simulink model "PID_model"  (R2020a)
settings: Solver=VariableStepAuto  StartTime=0.0  StopTime=10  RelTol=1e-3
values from neighbouring files (symbols this model uses):
  A = [0 0 0 1 0 0 0 0 0 0 0 0 ... (first row only)    [quadrotor_parameters.m]
  B = [0 0 0 0 ... (first row only)    [quadrotor_parameters.m]
  kf = 9.8e-6    (= 9.8e-06)    [quadrotor_parameters.m]
  km = 1.6e-7    (= 1.6e-07)    [quadrotor_parameters.m]
  w1 = 100    [quadrotor_parameters.m]
  w2 = 100    [quadrotor_parameters.m]
  w3 = 100    [quadrotor_parameters.m]
  w4 = 100    [quadrotor_parameters.m]
libraries: simulink x6
settings Model: Creator=Dr.Saraf  LastModifiedBy=Dr.Saraf
settings DataIOCC: ReturnWorkspaceOutputs=off
settings DebuggingCC: ArithmeticOperatorsInVariantConditions=warning
settings SFSimCC: SimUseLocalCustomCode=off  CustomCodeUndefinedFunction=UseInterfaceOnly
settings RTWCC: RTWUseLocalCustomCode=off
settings CodeAppCC: StateflowObjectComments=on

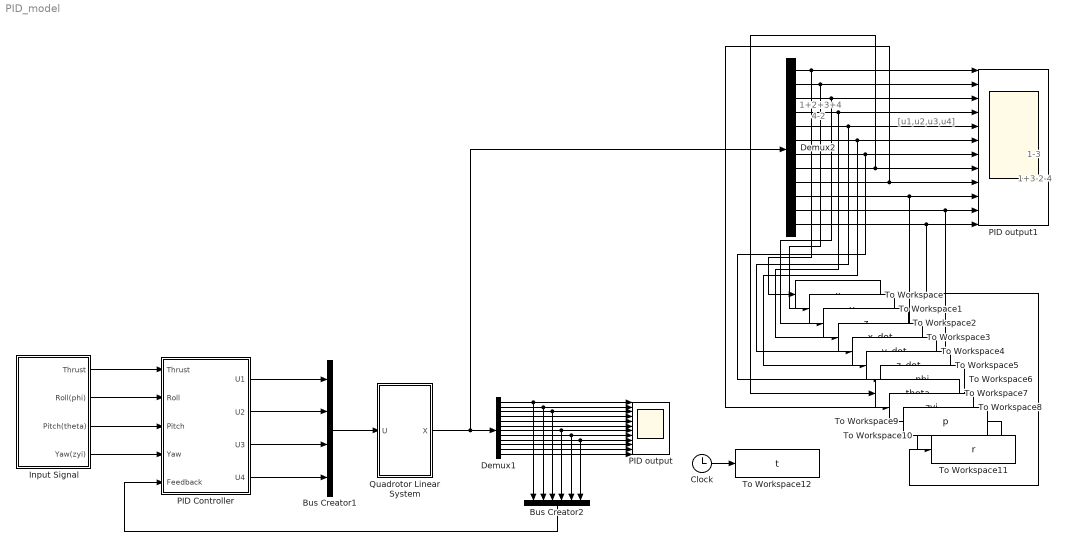
== system PID_model ==
  note: [u1,u2,u3,u4]
  note: 1+2+3+4
  note: 1+3-2-4
  note: 1-3
  note: 4-2
  Bus Creator1 : BusCreator  Inputs=4
  Bus Creator2 : BusCreator  Inputs=6
  Clock : Clock
  Demux1 : Demux  Outputs=12
  Demux2 : Demux  Outputs=12
  Input Signal : Subsystem
  PID Controller : Subsystem
  "PID output " : Scope  NumInputPorts=12
  "PID output1 " : Scope  NumInputPorts=12
  Quadrotor Linear System : Subsystem
  To Workspace : ToWorkspace  VariableName=x  SampleTime=0.1
  To Workspace1 : ToWorkspace  VariableName=y  SampleTime=0.1
  To Workspace10 : ToWorkspace  VariableName=q  SampleTime=0.001
  To Workspace11 : ToWorkspace  VariableName=r  SampleTime=0.001
  To Workspace12 : ToWorkspace  VariableName=t  SampleTime=0.001
  To Workspace2 : ToWorkspace  VariableName=z  SampleTime=0.1
  To Workspace3 : ToWorkspace  VariableName=x_dot  SampleTime=0.1
  To Workspace4 : ToWorkspace  VariableName=y_dot  SampleTime=0.1
  To Workspace5 : ToWorkspace  VariableName=z_dot  SampleTime=0.1
  To Workspace6 : ToWorkspace  VariableName=phi  SampleTime=0.001
  To Workspace7 : ToWorkspace  VariableName=theta  SampleTime=0.001
  To Workspace8 : ToWorkspace  VariableName=zyi  SampleTime=0.001
  To Workspace9 : ToWorkspace  VariableName=p  SampleTime=0.001
  wires:
  Demux1/5 -> "PID output "/5
  Demux1/11 -> "PID output "/11
  Demux1/12 -> "PID output "/12
  Demux1/4 -> "PID output "/4
  Demux1/10 -> "PID output "/10
  Demux1/6 -> "PID output "/6
  Demux1/1 -> "PID output "/1, Bus Creator2/1
  Demux1/9 -> "PID output "/9, Bus Creator2/6
  Demux1/7 -> "PID output "/7, Bus Creator2/4
  Demux1/3 -> "PID output "/3, Bus Creator2/3
  Demux1/8 -> "PID output "/8, Bus Creator2/5
  Demux1/2 -> "PID output "/2, Bus Creator2/2
  Bus Creator1/1 -> Quadrotor Linear System/1(U)
  Quadrotor Linear System/1(X) -> Demux2/1, Demux1/1
  Input Signal/1(Thrust) -> PID Controller/1(Thrust)
  Input Signal/2(Roll(phi)) -> PID Controller/2(Roll)
  Input Signal/3(Pitch(theta)) -> PID Controller/3(Pitch)
  Input Signal/4(Yaw(zyi)) -> PID Controller/4(Yaw)
  Bus Creator2/1 -> PID Controller/5(Feedback)
  PID Controller/1(U1) -> Bus Creator1/1
  PID Controller/2(U2) -> Bus Creator1/2
  PID Controller/3(U3) -> Bus Creator1/3
  PID Controller/4(U4) -> Bus Creator1/4
  Clock/1 -> To Workspace12/1
  Demux2/11 -> To Workspace10/1, "PID output1 "/11
  Demux2/5 -> To Workspace4/1, "PID output1 "/5
  Demux2/8 -> To Workspace7/1, "PID output1 "/8
  Demux2/10 -> To Workspace9/1, "PID output1 "/10
  Demux2/1 -> To Workspace/1, "PID output1 "/1
  Demux2/12 -> To Workspace11/1, "PID output1 "/12
  Demux2/3 -> To Workspace2/1, "PID output1 "/3
  Demux2/6 -> To Workspace5/1, "PID output1 "/6
  Demux2/9 -> To Workspace8/1, "PID output1 "/9
  Demux2/2 -> To Workspace1/1, "PID output1 "/2
  Demux2/4 -> To Workspace3/1, "PID output1 "/4
  Demux2/7 -> To Workspace6/1, "PID output1 "/7

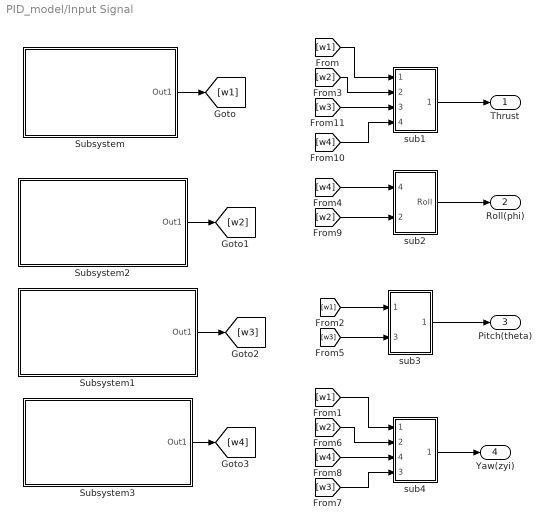
== system PID_model/Input Signal ==
  Subsystem : Subsystem
  Subsystem1 : Subsystem
  Subsystem2 : Subsystem
  Subsystem3 : Subsystem
  sub1 : Subsystem
  "sub2 " : Subsystem
  "sub3 " : Subsystem
  sub4 : Subsystem
  Thrust : Outport
  Roll(phi) : Outport  Port=2
  Pitch(theta) : Outport  Port=3
  Yaw(zyi) : Outport  Port=4
  wires:
  [w4] -> sub1/4(4)
  [w3] -> sub1/3(3)
  [w2] -> sub1/2(2)
  [w1] -> sub4/1(1)
  [w4] -> sub4/3("4 ")
  [w3] -> sub4/4("3 ")
  [w1] -> "sub3 "/1(1)
  [w4] -> "sub2 "/1(4)
  [w3] -> "sub3 "/2(3)
  [w1] -> sub1/1(1)
  [w2] -> sub4/2(2)
  [w2] -> "sub2 "/2(2)
  "sub2 "/1(Roll) -> Roll(phi)/1
  sub1/1(Thrust) -> Thrust/1
  sub4/1(Yaw) -> Yaw(zyi)/1
  "sub3 "/1(Pitch) -> Pitch(theta)/1
  Subsystem1/1(Out1) -> [w3]
  Subsystem/1(Out1) -> [w1]
  Subsystem2/1(Out1) -> [w2]
  Subsystem3/1(Out1) -> [w4]

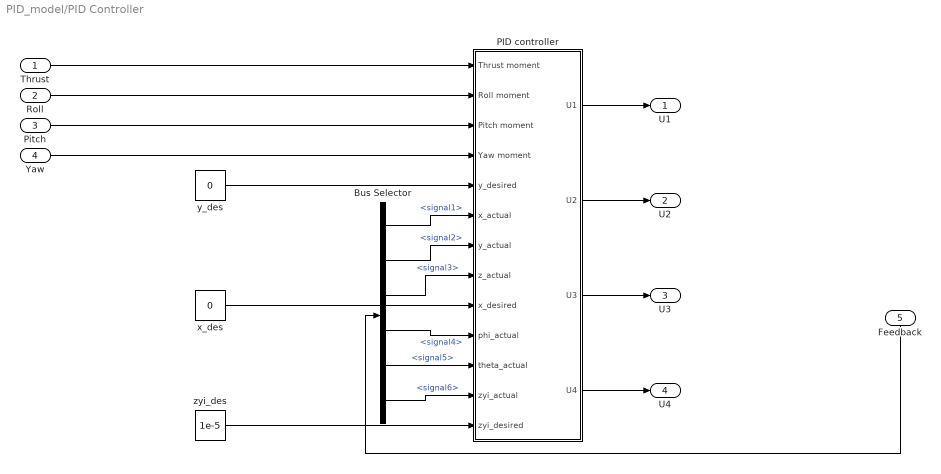
== system PID_model/PID Controller ==
  Thrust : Inport
  Roll : Inport  Port=2
  Pitch : Inport  Port=3
  Yaw : Inport  Port=4
  Feedback : Inport  Port=5
  Bus Selector : BusSelector  OutputSignals=signal1,signal2,signal3,signal4,signal5,signal6
  PID controller : Subsystem
  x_des : Constant  Value=0
  y_des : Constant  Value=0
  zyi_des : Constant  Value=1e-5
  U1 : Outport
  U2 : Outport  Port=2
  U3 : Outport  Port=3
  U4 : Outport  Port=4
  wires:
  Bus Selector/1 -> PID controller/6(x_actual)  "<signal1>"
  Thrust/1 -> PID controller/1(Thrust moment)
  Roll/1 -> PID controller/2(Roll moment)
  PID controller/3("U3 ") -> U3/1
  Bus Selector/2 -> PID controller/7(y_actual)  "<signal2>"
  x_des/1 -> PID controller/9(x_desired)
  zyi_des/1 -> PID controller/13(zyi_desired)
  Bus Selector/3 -> PID controller/8(z_actual)  "<signal3>"
  Bus Selector/6 -> PID controller/12(zyi_actual)  "<signal6>"
  Feedback/1 -> Bus Selector/1
  y_des/1 -> PID controller/5(y_desired)
  PID controller/2(U2) -> U2/1
  Yaw/1 -> PID controller/4(Yaw moment)
  Bus Selector/4 -> PID controller/10(phi_actual)  "<signal4>"
  PID controller/4(U4) -> U4/1
  Pitch/1 -> PID controller/3(Pitch moment)
  PID controller/1(U1) -> U1/1
  Bus Selector/5 -> PID controller/11(theta_actual)  "<signal5>"

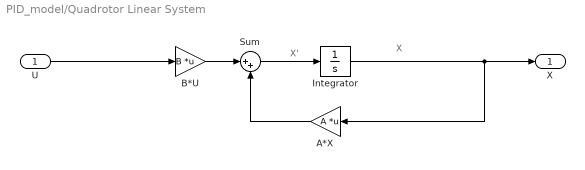
== system PID_model/Quadrotor Linear System ==
  note: X'
  note: X
  U : Inport
  A*X : Gain  Gain=A  Multiplication=Matrix(K*u)
  B*U : Gain  Gain=B  Multiplication=Matrix(K*u)
  Integrator : Integrator  InitialCondition=[1,1,1,1,1,1,1,1,1,1,1,1]
  Sum : Sum  Inputs=|++
  X : Outport
  wires:
  Integrator/1 -> X/1, A*X/1
  B*U/1 -> Sum/1
  Sum/1 -> Integrator/1
  A*X/1 -> Sum/2
  U/1 -> B*U/1

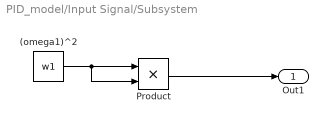
== system PID_model/Input Signal/Subsystem ==
  (omega1)^2 : Constant  Value=w1
  Product : Product
  Out1 : Outport
  wires:
  (omega1)^2/1 -> Product/2, Product/1
  Product/1 -> Out1/1

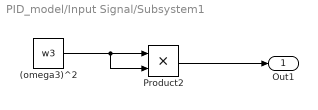
== system PID_model/Input Signal/Subsystem1 ==
  (omega3)^2 : Constant  Value=w3
  Product2 : Product
  Out1 : Outport
  wires:
  (omega3)^2/1 -> Product2/2, Product2/1
  Product2/1 -> Out1/1

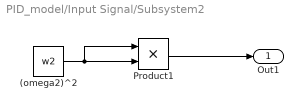
== system PID_model/Input Signal/Subsystem2 ==
  (omega2)^2 : Constant  Value=w2
  Product1 : Product
  Out1 : Outport
  wires:
  (omega2)^2/1 -> Product1/1, Product1/2
  Product1/1 -> Out1/1

== system PID_model/Input Signal/Subsystem3 ==
  (omega4)^2 : Constant  Value=w4
  Product3 : Product
  Out1 : Outport
  wires:
  (omega4)^2/1 -> Product3/2, Product3/1
  Product3/1 -> Out1/1

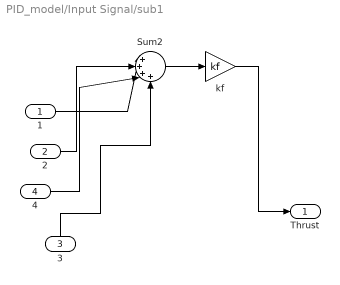
== system PID_model/Input Signal/sub1 ==
  1 : Inport
  2 : Inport  Port=2
  3 : Inport  Port=3
  4 : Inport  Port=4
  Sum2 : Sum  Inputs=|++++
  kf : Gain  Gain=kf
  Thrust : Outport
  wires:
  kf/1 -> Thrust/1
  Sum2/1 -> kf/1
  1/1 -> Sum2/1
  2/1 -> Sum2/2
  3/1 -> Sum2/4
  4/1 -> Sum2/3

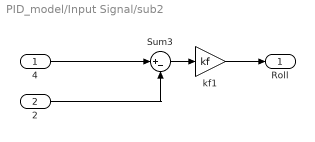
== system PID_model/Input Signal/sub2  ==
  4 : Inport
  2 : Inport  Port=2
  Sum3 : Sum  Inputs=|+-
  kf1 : Gain  Gain=kf
  Roll : Outport
  wires:
  kf1/1 -> Roll/1
  Sum3/1 -> kf1/1
  4/1 -> Sum3/1
  2/1 -> Sum3/2

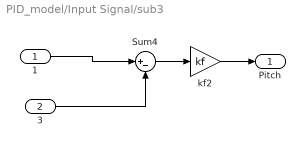
== system PID_model/Input Signal/sub3  ==
  1 : Inport
  3 : Inport  Port=2
  Sum4 : Sum  Inputs=|+-
  kf2 : Gain  Gain=kf
  Pitch : Outport
  wires:
  3/1 -> Sum4/2
  1/1 -> Sum4/1
  Sum4/1 -> kf2/1
  kf2/1 -> Pitch/1

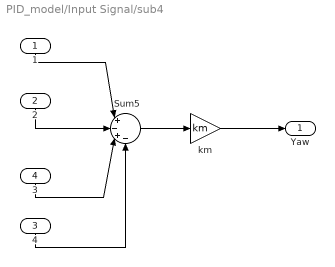
== system PID_model/Input Signal/sub4 ==
  1 : Inport
  2 : Inport  Port=2
  "4 " : Inport  Port=3
  "3 " : Inport  Port=4
  Sum5 : Sum  Inputs=|+-+-
  km : Gain  Gain=km
  Yaw : Outport
  wires:
  Sum5/1 -> km/1
  km/1 -> Yaw/1
  "3 "/1 -> Sum5/3
  2/1 -> Sum5/2
  "4 "/1 -> Sum5/4
  1/1 -> Sum5/1

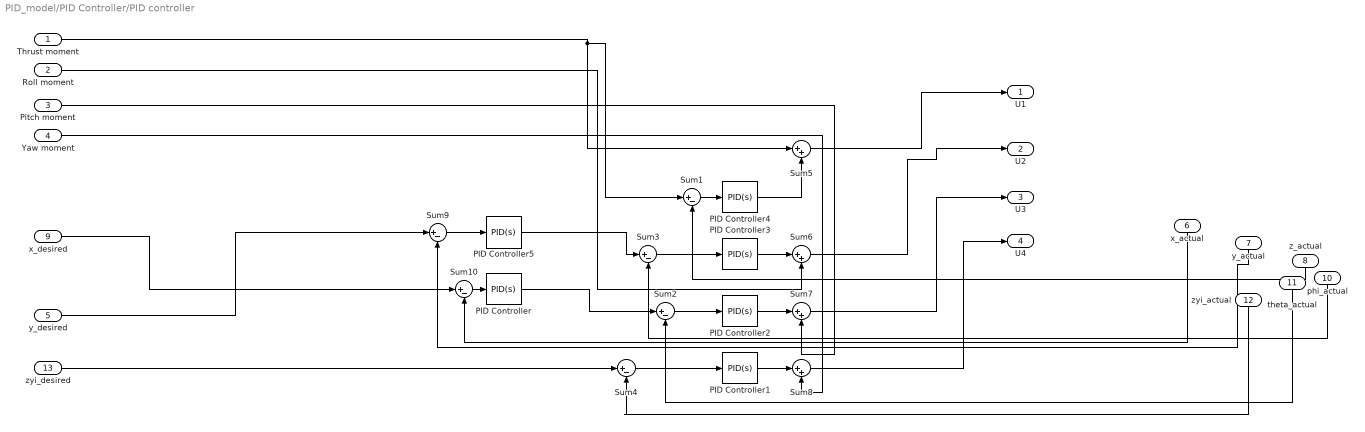
== system PID_model/PID Controller/PID controller ==
  Thrust moment : Inport
  Roll moment : Inport  Port=2
  Pitch moment : Inport  Port=3
  Yaw moment : Inport  Port=4
  y_desired : Inport  Port=5
  x_actual : Inport  Port=6
  y_actual : Inport  Port=7
  z_actual : Inport  Port=8
  x_desired : Inport  Port=9
  phi_actual : Inport  Port=10
  theta_actual : Inport  Port=11
  zyi_actual : Inport  Port=12
  zyi_desired : Inport  Port=13
  PID Controller : simulink/Continuous/PID Controller  Controller=PID  Form=Parallel  TimeDomain=Continuous-time  UseExternalTs=off  SampleTime=-1  IntegratorMethod=Forward Euler  FilterMethod=Forward Euler  ControllerParametersSource=internal  P=2.93760850093011  I=0.0320571710777629  D=4.86506551746036  UseFilter=on  N=2.18607719154356  TunerSelectOption=Transfer Function Based (PID Tuner App)  InitialConditionSource=internal  InitialConditionForIntegrator=0  InitialConditionForFilter=0  DifferentiatorICPrevScaledInput=0  ExternalReset=none  TrackingMode=off  Kt=1  LimitOutput=off  UpperSaturationLimit=inf  LowerSaturationLimit=-inf  LinearizeAsGain=on  AntiWindupMode=none  Kb=1  POutMin=[]  POutMax=[]  IOutMin=[]  IOutMax=[]  DOutMin=[]  DOutMax=[]  NOutMin=[]  NOutMax=[]  SumOutMin=[]  SumOutMax=[]  SaturationOutMin=[]  SaturationOutMax=[]  PParamMin=[]  PParamMax=[]  IParamMin=[]  IParamMax=[]  DParamMin=[]  DParamMax=[]  NParamMin=[]  NParamMax=[]  KbParamMin=[]  KbParamMax=[]  KtParamMin=[]  KtParamMax=[]  KbOutMin=[]  KbOutMax=[]  KtOutMin=[]  KtOutMax=[]  IntegratorOutMin=[]  IntegratorOutMax=[]  FilterOutMin=[]  FilterOutMax=[]  SumI1OutMin=[]  SumI1OutMax=[]  SumI2OutMin=[]  SumI2OutMax=[]  SumI3OutMin=[]  SumI3OutMax=[]  SumI4OutMin=[]  SumI4OutMax=[]  SumDOutMin=[]  SumDOutMax=[]  DifferentiatorOutMin=[]  DifferentiatorOutMax=[]  FilterDiffOutCoefMin=[]  FilterDiffOutCoefMax=[]  ReciprocalOutMin=[]  ReciprocalOutMax=[]  SumDenOutMin=[]  SumDenOutMax=[]  SumNumOutMin=[]  SumNumOutMax=[]  DivideOutMin=[]  DivideOutMax=[]  UdiffTsProdOutMin=[]  UdiffTsProdOutMax=[]  NTsProdOutMin=[]  NTsProdOutMax=[]  UintegralTsProdOutMin=[]  UintegralTsProdOutMax=[]  UngainTsProdOutMin=[]  UngainTsProdOutMax=[]  IntegratorContinuousStateAttributes=''  IntegratorStateMustResolveToSignalObject=off  IntegratorRTWStateStorageClass=Auto  FilterContinuousStateAttributes=''  FilterStateMustResolveToSignalObject=off  FilterRTWStateStorageClass=Auto  ParallelPVariant=InternalParameters  IdealPVariant=Disabled  IVariant=InternalParameters  DVariant=InternalParameters  IntegratorVariant=Continuous  SatVariant=Disabled  AWVariant=Passthrough  PCopyVariant=Disabled  TRVariant=Disabled  FdbkBlocksVariant=Forward  IdealPFdbkVariant=Disabled  SatFdbkVariant=Disabled  DerivativeFilterVariant=ContFilter  NVariant=InternalParameters  NCopyVariant=Disabled  FilterICVariant=InternalICsFilter  IntegratorICVariant=InternalICs  ExternalResetVariant=Disabled  TRSumVariant=Passthrough  SumFdbkVariant=Disabled  SumVariant=Sum_PID  TsampFilterVariant=InternalTs  TsampNgainVariant=Passthrough  TsampIntegralVariant=Passthrough
  PID Controller1 : simulink/Continuous/PID Controller  Controller=PID  Form=Parallel  TimeDomain=Continuous-time  UseExternalTs=off  SampleTime=-1  IntegratorMethod=Forward Euler  FilterMethod=Forward Euler  ControllerParametersSource=internal  P=0.0131233252055703  I=0.000765605460811457  D=0.0499808607427746  UseFilter=on  N=1142.8279760416  TunerSelectOption=Transfer Function Based (PID Tuner App)  InitialConditionSource=internal  InitialConditionForIntegrator=0  InitialConditionForFilter=0  DifferentiatorICPrevScaledInput=0  ExternalReset=none  TrackingMode=off  Kt=1  LimitOutput=off  UpperSaturationLimit=inf  LowerSaturationLimit=-inf  LinearizeAsGain=on  AntiWindupMode=none  Kb=1  POutMin=[]  POutMax=[]  IOutMin=[]  IOutMax=[]  DOutMin=[]  DOutMax=[]  NOutMin=[]  NOutMax=[]  SumOutMin=[]  SumOutMax=[]  SaturationOutMin=[]  SaturationOutMax=[]  PParamMin=[]  PParamMax=[]  IParamMin=[]  IParamMax=[]  DParamMin=[]  DParamMax=[]  NParamMin=[]  NParamMax=[]  KbParamMin=[]  KbParamMax=[]  KtParamMin=[]  KtParamMax=[]  KbOutMin=[]  KbOutMax=[]  KtOutMin=[]  KtOutMax=[]  IntegratorOutMin=[]  IntegratorOutMax=[]  FilterOutMin=[]  FilterOutMax=[]  SumI1OutMin=[]  SumI1OutMax=[]  SumI2OutMin=[]  SumI2OutMax=[]  SumI3OutMin=[]  SumI3OutMax=[]  SumI4OutMin=[]  SumI4OutMax=[]  SumDOutMin=[]  SumDOutMax=[]  DifferentiatorOutMin=[]  DifferentiatorOutMax=[]  FilterDiffOutCoefMin=[]  FilterDiffOutCoefMax=[]  ReciprocalOutMin=[]  ReciprocalOutMax=[]  SumDenOutMin=[]  SumDenOutMax=[]  SumNumOutMin=[]  SumNumOutMax=[]  DivideOutMin=[]  DivideOutMax=[]  UdiffTsProdOutMin=[]  UdiffTsProdOutMax=[]  NTsProdOutMin=[]  NTsProdOutMax=[]  UintegralTsProdOutMin=[]  UintegralTsProdOutMax=[]  UngainTsProdOutMin=[]  UngainTsProdOutMax=[]  IntegratorContinuousStateAttributes=''  IntegratorStateMustResolveToSignalObject=off  IntegratorRTWStateStorageClass=Auto  FilterContinuousStateAttributes=''  FilterStateMustResolveToSignalObject=off  FilterRTWStateStorageClass=Auto  ParallelPVariant=InternalParameters  IdealPVariant=Disabled  IVariant=InternalParameters  DVariant=InternalParameters  IntegratorVariant=Continuous  SatVariant=Disabled  AWVariant=Passthrough  PCopyVariant=Disabled  TRVariant=Disabled  FdbkBlocksVariant=Forward  IdealPFdbkVariant=Disabled  SatFdbkVariant=Disabled  DerivativeFilterVariant=ContFilter  NVariant=InternalParameters  NCopyVariant=Disabled  FilterICVariant=InternalICsFilter  IntegratorICVariant=InternalICs  ExternalResetVariant=Disabled  TRSumVariant=Passthrough  SumFdbkVariant=Disabled  SumVariant=Sum_PID  TsampFilterVariant=InternalTs  TsampNgainVariant=Passthrough  TsampIntegralVariant=Passthrough
  PID Controller2 : simulink/Continuous/PID Controller  Controller=PID  Form=Parallel  TimeDomain=Continuous-time  UseExternalTs=off  SampleTime=-1  IntegratorMethod=Forward Euler  FilterMethod=Forward Euler  ControllerParametersSource=internal  P=4.03605230374903  I=10.0303452891104  D=0.326387790675753  UseFilter=on  N=96.1522448129433  TunerSelectOption=Transfer Function Based (PID Tuner App)  InitialConditionSource=internal  InitialConditionForIntegrator=0  InitialConditionForFilter=0  DifferentiatorICPrevScaledInput=0  ExternalReset=none  TrackingMode=off  Kt=1  LimitOutput=off  UpperSaturationLimit=inf  LowerSaturationLimit=-inf  LinearizeAsGain=on  AntiWindupMode=none  Kb=1  POutMin=[]  POutMax=[]  IOutMin=[]  IOutMax=[]  DOutMin=[]  DOutMax=[]  NOutMin=[]  NOutMax=[]  SumOutMin=[]  SumOutMax=[]  SaturationOutMin=[]  SaturationOutMax=[]  PParamMin=[]  PParamMax=[]  IParamMin=[]  IParamMax=[]  DParamMin=[]  DParamMax=[]  NParamMin=[]  NParamMax=[]  KbParamMin=[]  KbParamMax=[]  KtParamMin=[]  KtParamMax=[]  KbOutMin=[]  KbOutMax=[]  KtOutMin=[]  KtOutMax=[]  IntegratorOutMin=[]  IntegratorOutMax=[]  FilterOutMin=[]  FilterOutMax=[]  SumI1OutMin=[]  SumI1OutMax=[]  SumI2OutMin=[]  SumI2OutMax=[]  SumI3OutMin=[]  SumI3OutMax=[]  SumI4OutMin=[]  SumI4OutMax=[]  SumDOutMin=[]  SumDOutMax=[]  DifferentiatorOutMin=[]  DifferentiatorOutMax=[]  FilterDiffOutCoefMin=[]  FilterDiffOutCoefMax=[]  ReciprocalOutMin=[]  ReciprocalOutMax=[]  SumDenOutMin=[]  SumDenOutMax=[]  SumNumOutMin=[]  SumNumOutMax=[]  DivideOutMin=[]  DivideOutMax=[]  UdiffTsProdOutMin=[]  UdiffTsProdOutMax=[]  NTsProdOutMin=[]  NTsProdOutMax=[]  UintegralTsProdOutMin=[]  UintegralTsProdOutMax=[]  UngainTsProdOutMin=[]  UngainTsProdOutMax=[]  IntegratorContinuousStateAttributes=''  IntegratorStateMustResolveToSignalObject=off  IntegratorRTWStateStorageClass=Auto  FilterContinuousStateAttributes=''  FilterStateMustResolveToSignalObject=off  FilterRTWStateStorageClass=Auto  ParallelPVariant=InternalParameters  IdealPVariant=Disabled  IVariant=InternalParameters  DVariant=InternalParameters  IntegratorVariant=Continuous  SatVariant=Disabled  AWVariant=Passthrough  PCopyVariant=Disabled  TRVariant=Disabled  FdbkBlocksVariant=Forward  IdealPFdbkVariant=Disabled  SatFdbkVariant=Disabled  DerivativeFilterVariant=ContFilter  NVariant=InternalParameters  NCopyVariant=Disabled  FilterICVariant=InternalICsFilter  IntegratorICVariant=InternalICs  ExternalResetVariant=Disabled  TRSumVariant=Passthrough  SumFdbkVariant=Disabled  SumVariant=Sum_PID  TsampFilterVariant=InternalTs  TsampNgainVariant=Passthrough  TsampIntegralVariant=Passthrough
  PID Controller3 : simulink/Continuous/PID Controller  Controller=PID  Form=Parallel  TimeDomain=Continuous-time  UseExternalTs=off  SampleTime=-1  IntegratorMethod=Forward Euler  FilterMethod=Forward Euler  ControllerParametersSource=internal  P=4.03693263836556  I=10.0343260984356  D=0.326415540304519  UseFilter=on  N=96.1610558780663  TunerSelectOption=Transfer Function Based (PID Tuner App)  InitialConditionSource=internal  InitialConditionForIntegrator=0  InitialConditionForFilter=0  DifferentiatorICPrevScaledInput=0  ExternalReset=none  TrackingMode=off  Kt=1  LimitOutput=off  UpperSaturationLimit=inf  LowerSaturationLimit=-inf  LinearizeAsGain=on  AntiWindupMode=none  Kb=1  POutMin=[]  POutMax=[]  IOutMin=[]  IOutMax=[]  DOutMin=[]  DOutMax=[]  NOutMin=[]  NOutMax=[]  SumOutMin=[]  SumOutMax=[]  SaturationOutMin=[]  SaturationOutMax=[]  PParamMin=[]  PParamMax=[]  IParamMin=[]  IParamMax=[]  DParamMin=[]  DParamMax=[]  NParamMin=[]  NParamMax=[]  KbParamMin=[]  KbParamMax=[]  KtParamMin=[]  KtParamMax=[]  KbOutMin=[]  KbOutMax=[]  KtOutMin=[]  KtOutMax=[]  IntegratorOutMin=[]  IntegratorOutMax=[]  FilterOutMin=[]  FilterOutMax=[]  SumI1OutMin=[]  SumI1OutMax=[]  SumI2OutMin=[]  SumI2OutMax=[]  SumI3OutMin=[]  SumI3OutMax=[]  SumI4OutMin=[]  SumI4OutMax=[]  SumDOutMin=[]  SumDOutMax=[]  DifferentiatorOutMin=[]  DifferentiatorOutMax=[]  FilterDiffOutCoefMin=[]  FilterDiffOutCoefMax=[]  ReciprocalOutMin=[]  ReciprocalOutMax=[]  SumDenOutMin=[]  SumDenOutMax=[]  SumNumOutMin=[]  SumNumOutMax=[]  DivideOutMin=[]  DivideOutMax=[]  UdiffTsProdOutMin=[]  UdiffTsProdOutMax=[]  NTsProdOutMin=[]  NTsProdOutMax=[]  UintegralTsProdOutMin=[]  UintegralTsProdOutMax=[]  UngainTsProdOutMin=[]  UngainTsProdOutMax=[]  IntegratorContinuousStateAttributes=''  IntegratorStateMustResolveToSignalObject=off  IntegratorRTWStateStorageClass=Auto  FilterContinuousStateAttributes=''  FilterStateMustResolveToSignalObject=off  FilterRTWStateStorageClass=Auto  ParallelPVariant=InternalParameters  IdealPVariant=Disabled  IVariant=InternalParameters  DVariant=InternalParameters  IntegratorVariant=Continuous  SatVariant=Disabled  AWVariant=Passthrough  PCopyVariant=Disabled  TRVariant=Disabled  FdbkBlocksVariant=Forward  IdealPFdbkVariant=Disabled  SatFdbkVariant=Disabled  DerivativeFilterVariant=ContFilter  NVariant=InternalParameters  NCopyVariant=Disabled  FilterICVariant=InternalICsFilter  IntegratorICVariant=InternalICs  ExternalResetVariant=Disabled  TRSumVariant=Passthrough  SumFdbkVariant=Disabled  SumVariant=Sum_PID  TsampFilterVariant=InternalTs  TsampNgainVariant=Passthrough  TsampIntegralVariant=Passthrough
  PID Controller4 : simulink/Continuous/PID Controller  Controller=PID  Form=Parallel  TimeDomain=Continuous-time  UseExternalTs=off  SampleTime=-1  IntegratorMethod=Forward Euler  FilterMethod=Forward Euler  ControllerParametersSource=internal  P=9.09174597457637  I=1.94133684655557  D=10.4078264490623  UseFilter=on  N=599.764647608782  TunerSelectOption=Transfer Function Based (PID Tuner App)  InitialConditionSource=internal  InitialConditionForIntegrator=0  InitialConditionForFilter=0  DifferentiatorICPrevScaledInput=0  ExternalReset=none  TrackingMode=off  Kt=1  LimitOutput=off  UpperSaturationLimit=inf  LowerSaturationLimit=-inf  LinearizeAsGain=on  AntiWindupMode=none  Kb=1  POutMin=[]  POutMax=[]  IOutMin=[]  IOutMax=[]  DOutMin=[]  DOutMax=[]  NOutMin=[]  NOutMax=[]  SumOutMin=[]  SumOutMax=[]  SaturationOutMin=[]  SaturationOutMax=[]  PParamMin=[]  PParamMax=[]  IParamMin=[]  IParamMax=[]  DParamMin=[]  DParamMax=[]  NParamMin=[]  NParamMax=[]  KbParamMin=[]  KbParamMax=[]  KtParamMin=[]  KtParamMax=[]  KbOutMin=[]  KbOutMax=[]  KtOutMin=[]  KtOutMax=[]  IntegratorOutMin=[]  IntegratorOutMax=[]  FilterOutMin=[]  FilterOutMax=[]  SumI1OutMin=[]  SumI1OutMax=[]  SumI2OutMin=[]  SumI2OutMax=[]  SumI3OutMin=[]  SumI3OutMax=[]  SumI4OutMin=[]  SumI4OutMax=[]  SumDOutMin=[]  SumDOutMax=[]  DifferentiatorOutMin=[]  DifferentiatorOutMax=[]  FilterDiffOutCoefMin=[]  FilterDiffOutCoefMax=[]  ReciprocalOutMin=[]  ReciprocalOutMax=[]  SumDenOutMin=[]  SumDenOutMax=[]  SumNumOutMin=[]  SumNumOutMax=[]  DivideOutMin=[]  DivideOutMax=[]  UdiffTsProdOutMin=[]  UdiffTsProdOutMax=[]  NTsProdOutMin=[]  NTsProdOutMax=[]  UintegralTsProdOutMin=[]  UintegralTsProdOutMax=[]  UngainTsProdOutMin=[]  UngainTsProdOutMax=[]  IntegratorContinuousStateAttributes=''  IntegratorStateMustResolveToSignalObject=off  IntegratorRTWStateStorageClass=Auto  FilterContinuousStateAttributes=''  FilterStateMustResolveToSignalObject=off  FilterRTWStateStorageClass=Auto  ParallelPVariant=InternalParameters  IdealPVariant=Disabled  IVariant=InternalParameters  DVariant=InternalParameters  IntegratorVariant=Continuous  SatVariant=Disabled  AWVariant=Passthrough  PCopyVariant=Disabled  TRVariant=Disabled  FdbkBlocksVariant=Forward  IdealPFdbkVariant=Disabled  SatFdbkVariant=Disabled  DerivativeFilterVariant=ContFilter  NVariant=InternalParameters  NCopyVariant=Disabled  FilterICVariant=InternalICsFilter  IntegratorICVariant=InternalICs  ExternalResetVariant=Disabled  TRSumVariant=Passthrough  SumFdbkVariant=Disabled  SumVariant=Sum_PID  TsampFilterVariant=InternalTs  TsampNgainVariant=Passthrough  TsampIntegralVariant=Passthrough
  PID Controller5 : simulink/Continuous/PID Controller  Controller=PID  Form=Parallel  TimeDomain=Continuous-time  UseExternalTs=off  SampleTime=-1  IntegratorMethod=Forward Euler  FilterMethod=Forward Euler  ControllerParametersSource=internal  P=-2.92765548051597  I=-0.0319622087005284  D=-4.67579680459697  UseFilter=on  N=2.18553276928718  TunerSelectOption=Transfer Function Based (PID Tuner App)  InitialConditionSource=internal  InitialConditionForIntegrator=0  InitialConditionForFilter=0  DifferentiatorICPrevScaledInput=0  ExternalReset=none  TrackingMode=off  Kt=1  LimitOutput=off  UpperSaturationLimit=inf  LowerSaturationLimit=-inf  LinearizeAsGain=on  AntiWindupMode=none  Kb=1  POutMin=[]  POutMax=[]  IOutMin=[]  IOutMax=[]  DOutMin=[]  DOutMax=[]  NOutMin=[]  NOutMax=[]  SumOutMin=[]  SumOutMax=[]  SaturationOutMin=[]  SaturationOutMax=[]  PParamMin=[]  PParamMax=[]  IParamMin=[]  IParamMax=[]  DParamMin=[]  DParamMax=[]  NParamMin=[]  NParamMax=[]  KbParamMin=[]  KbParamMax=[]  KtParamMin=[]  KtParamMax=[]  KbOutMin=[]  KbOutMax=[]  KtOutMin=[]  KtOutMax=[]  IntegratorOutMin=[]  IntegratorOutMax=[]  FilterOutMin=[]  FilterOutMax=[]  SumI1OutMin=[]  SumI1OutMax=[]  SumI2OutMin=[]  SumI2OutMax=[]  SumI3OutMin=[]  SumI3OutMax=[]  SumI4OutMin=[]  SumI4OutMax=[]  SumDOutMin=[]  SumDOutMax=[]  DifferentiatorOutMin=[]  DifferentiatorOutMax=[]  FilterDiffOutCoefMin=[]  FilterDiffOutCoefMax=[]  ReciprocalOutMin=[]  ReciprocalOutMax=[]  SumDenOutMin=[]  SumDenOutMax=[]  SumNumOutMin=[]  SumNumOutMax=[]  DivideOutMin=[]  DivideOutMax=[]  UdiffTsProdOutMin=[]  UdiffTsProdOutMax=[]  NTsProdOutMin=[]  NTsProdOutMax=[]  UintegralTsProdOutMin=[]  UintegralTsProdOutMax=[]  UngainTsProdOutMin=[]  UngainTsProdOutMax=[]  IntegratorContinuousStateAttributes=''  IntegratorStateMustResolveToSignalObject=off  IntegratorRTWStateStorageClass=Auto  FilterContinuousStateAttributes=''  FilterStateMustResolveToSignalObject=off  FilterRTWStateStorageClass=Auto  ParallelPVariant=InternalParameters  IdealPVariant=Disabled  IVariant=InternalParameters  DVariant=InternalParameters  IntegratorVariant=Continuous  SatVariant=Disabled  AWVariant=Passthrough  PCopyVariant=Disabled  TRVariant=Disabled  FdbkBlocksVariant=Forward  IdealPFdbkVariant=Disabled  SatFdbkVariant=Disabled  DerivativeFilterVariant=ContFilter  NVariant=InternalParameters  NCopyVariant=Disabled  FilterICVariant=InternalICsFilter  IntegratorICVariant=InternalICs  ExternalResetVariant=Disabled  TRSumVariant=Passthrough  SumFdbkVariant=Disabled  SumVariant=Sum_PID  TsampFilterVariant=InternalTs  TsampNgainVariant=Passthrough  TsampIntegralVariant=Passthrough
  Sum{1..4,9..10} (6 alike) : Sum  Inputs=|+-
  Sum{5..8} (4 alike) : Sum  Inputs=|++
  U1 : Outport
  U2 : Outport  Port=2
  "U3 " : Outport  Port=3
  U4 : Outport  Port=4
  wires:
  Sum2/1 -> PID Controller2/1
  Pitch moment/1 -> Sum7/2
  Sum3/1 -> PID Controller3/1
  Roll moment/1 -> Sum6/2
  x_desired/1 -> Sum10/1
  Sum1/1 -> PID Controller4/1
  Sum4/1 -> PID Controller1/1
  Yaw moment/1 -> Sum8/2
  PID Controller4/1 -> Sum5/2
  PID Controller1/1 -> Sum8/1
  Thrust moment/1 -> Sum1/1, Sum5/1
  PID Controller2/1 -> Sum7/1
  Sum5/1 -> U1/1
  PID Controller5/1 -> Sum3/1
  Sum7/1 -> "U3 "/1
  Sum8/1 -> U4/1
  Sum6/1 -> U2/1
  Sum10/1 -> PID Controller/1
  y_actual/1 -> Sum9/2
  zyi_actual/1 -> Sum4/2
  phi_actual/1 -> Sum3/2
  z_actual/1 -> Sum1/2
  theta_actual/1 -> Sum2/2
  x_actual/1 -> Sum10/2
  Sum9/1 -> PID Controller5/1
  y_desired/1 -> Sum9/1
  PID Controller/1 -> Sum2/1
  zyi_desired/1 -> Sum4/1
  PID Controller3/1 -> Sum6/1
